simulink model "Q3"  (R2019a)
settings: Solver=FixedStepAuto  StartTime=0.0  StopTime=simulation_stop_time  RelTol=1e-3
values from neighbouring files (symbols this model uses):
  sample_time = 1 / input_sample_freq    (= 1e-06)    [testbench_Q1.m]    (also in testbench_Q3.m; testbench_Q5.m)
libraries: simulink x2
settings Model: Creator=qurai  LastModifiedBy=ASUAD\sasiddi8
settings OptimizationCC: BlockReduction=off  ConditionallyExecuteInputs=off  DefaultParameterBehavior=Inlined
settings DebuggingCC: AlgebraicLoopMsg=error
settings HardwareCC: ProdBitPerPointer=32  ProdBitPerSizeT=32  ProdBitPerPtrDiffT=32  ProdLargestAtomicFloat=None  ProdIntDivRoundTo=Undefined  ProdEndianess=Unspecified  ProdWordSize=32  ProdHWDeviceType=ASIC/FPGA->ASIC/FPGA  TargetBitPerLong=64  TargetBitPerPointer=64  TargetBitPerSizeT=64  TargetBitPerPtrDiffT=64  TargetLongLongMode=on  TargetIntDivRoundTo=Zero  TargetEndianess=LittleEndian  TargetWordSize=64  TargetHWDeviceType=Custom Processor->MATLAB Host Computer  ProdEqTarget=off

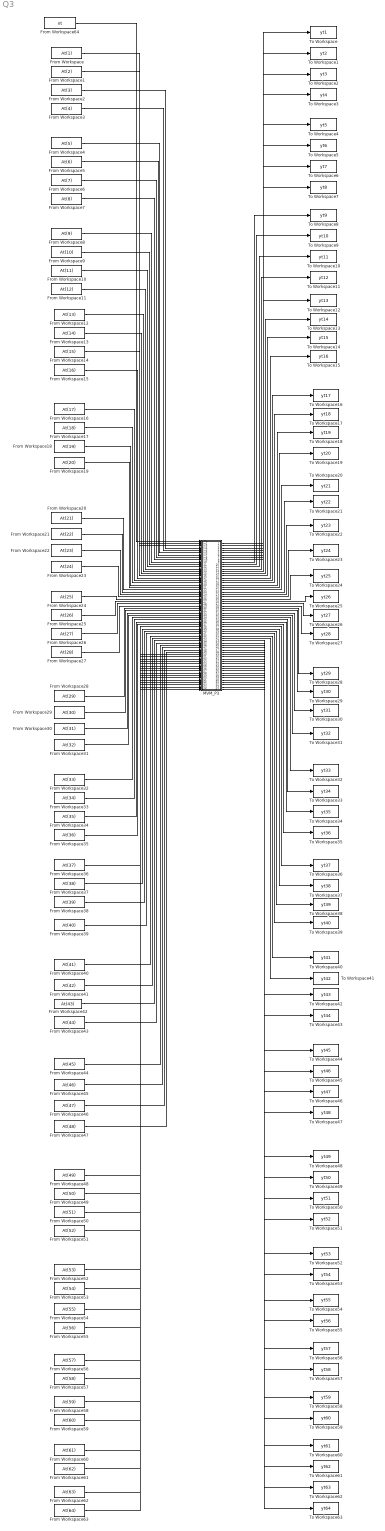
== system Q3 ==
  From Workspace : FromWorkspace  VariableName=At(1)  Interpolate=off  OutputAfterFinalValue=Holding final value
  From Workspace1 : FromWorkspace  VariableName=At(2)  Interpolate=off  OutputAfterFinalValue=Holding final value
  From Workspace10 : FromWorkspace  VariableName=At(11)  Interpolate=off  OutputAfterFinalValue=Holding final value
  From Workspace11 : FromWorkspace  VariableName=At(12)  Interpolate=off  OutputAfterFinalValue=Holding final value
  From Workspace12 : FromWorkspace  VariableName=At(13)  Interpolate=off  OutputAfterFinalValue=Holding final value
  From Workspace13 : FromWorkspace  VariableName=At(14)  Interpolate=off  OutputAfterFinalValue=Holding final value
  From Workspace14 : FromWorkspace  VariableName=At(15)  Interpolate=off  OutputAfterFinalValue=Holding final value
  From Workspace15 : FromWorkspace  VariableName=At(16)  Interpolate=off  OutputAfterFinalValue=Holding final value
  From Workspace16 : FromWorkspace  VariableName=At(17)  Interpolate=off  OutputAfterFinalValue=Holding final value
  From Workspace17 : FromWorkspace  VariableName=At(18)  Interpolate=off  OutputAfterFinalValue=Holding final value
  From Workspace18 : FromWorkspace  VariableName=At(19)  Interpolate=off  OutputAfterFinalValue=Holding final value
  From Workspace19 : FromWorkspace  VariableName=At(20)  Interpolate=off  OutputAfterFinalValue=Holding final value
  From Workspace2 : FromWorkspace  VariableName=At(3)  Interpolate=off  OutputAfterFinalValue=Holding final value
  From Workspace20 : FromWorkspace  VariableName=At(21)  Interpolate=off  OutputAfterFinalValue=Holding final value
  From Workspace21 : FromWorkspace  VariableName=At(22)  Interpolate=off  OutputAfterFinalValue=Holding final value
  From Workspace22 : FromWorkspace  VariableName=At(23)  Interpolate=off  OutputAfterFinalValue=Holding final value
  From Workspace23 : FromWorkspace  VariableName=At(24)  Interpolate=off  OutputAfterFinalValue=Holding final value
  From Workspace24 : FromWorkspace  VariableName=At(25)  Interpolate=off  OutputAfterFinalValue=Holding final value
  From Workspace25 : FromWorkspace  VariableName=At(26)  Interpolate=off  OutputAfterFinalValue=Holding final value
  From Workspace26 : FromWorkspace  VariableName=At(27)  Interpolate=off  OutputAfterFinalValue=Holding final value
  From Workspace27 : FromWorkspace  VariableName=At(28)  Interpolate=off  OutputAfterFinalValue=Holding final value
  From Workspace28 : FromWorkspace  VariableName=At(29)  Interpolate=off  OutputAfterFinalValue=Holding final value
  From Workspace29 : FromWorkspace  VariableName=At(30)  Interpolate=off  OutputAfterFinalValue=Holding final value
  From Workspace3 : FromWorkspace  VariableName=At(4)  Interpolate=off  OutputAfterFinalValue=Holding final value
  From Workspace30 : FromWorkspace  VariableName=At(31)  Interpolate=off  OutputAfterFinalValue=Holding final value
  From Workspace31 : FromWorkspace  VariableName=At(32)  Interpolate=off  OutputAfterFinalValue=Holding final value
  From Workspace32 : FromWorkspace  VariableName=At(33)  Interpolate=off  OutputAfterFinalValue=Holding final value
  From Workspace33 : FromWorkspace  VariableName=At(34)  Interpolate=off  OutputAfterFinalValue=Holding final value
  From Workspace34 : FromWorkspace  VariableName=At(35)  Interpolate=off  OutputAfterFinalValue=Holding final value
  From Workspace35 : FromWorkspace  VariableName=At(36)  Interpolate=off  OutputAfterFinalValue=Holding final value
  From Workspace36 : FromWorkspace  VariableName=At(37)  Interpolate=off  OutputAfterFinalValue=Holding final value
  From Workspace37 : FromWorkspace  VariableName=At(38)  Interpolate=off  OutputAfterFinalValue=Holding final value
  From Workspace38 : FromWorkspace  VariableName=At(39)  Interpolate=off  OutputAfterFinalValue=Holding final value
  From Workspace39 : FromWorkspace  VariableName=At(40)  Interpolate=off  OutputAfterFinalValue=Holding final value
  From Workspace4 : FromWorkspace  VariableName=At(5)  Interpolate=off  OutputAfterFinalValue=Holding final value
  From Workspace40 : FromWorkspace  VariableName=At(41)  Interpolate=off  OutputAfterFinalValue=Holding final value
  From Workspace41 : FromWorkspace  VariableName=At(42)  Interpolate=off  OutputAfterFinalValue=Holding final value
  From Workspace42 : FromWorkspace  VariableName=At(43)  Interpolate=off  OutputAfterFinalValue=Holding final value
  From Workspace43 : FromWorkspace  VariableName=At(44)  Interpolate=off  OutputAfterFinalValue=Holding final value
  From Workspace44 : FromWorkspace  VariableName=At(45)  Interpolate=off  OutputAfterFinalValue=Holding final value
  From Workspace45 : FromWorkspace  VariableName=At(46)  Interpolate=off  OutputAfterFinalValue=Holding final value
  From Workspace46 : FromWorkspace  VariableName=At(47)  Interpolate=off  OutputAfterFinalValue=Holding final value
  From Workspace47 : FromWorkspace  VariableName=At(48)  Interpolate=off  OutputAfterFinalValue=Holding final value
  From Workspace48 : FromWorkspace  VariableName=At(49)  Interpolate=off  OutputAfterFinalValue=Holding final value
  From Workspace49 : FromWorkspace  VariableName=At(50)  Interpolate=off  OutputAfterFinalValue=Holding final value
  From Workspace5 : FromWorkspace  VariableName=At(6)  Interpolate=off  OutputAfterFinalValue=Holding final value
  From Workspace50 : FromWorkspace  VariableName=At(51)  Interpolate=off  OutputAfterFinalValue=Holding final value
  From Workspace51 : FromWorkspace  VariableName=At(52)  Interpolate=off  OutputAfterFinalValue=Holding final value
  From Workspace52 : FromWorkspace  VariableName=At(53)  Interpolate=off  OutputAfterFinalValue=Holding final value
  From Workspace53 : FromWorkspace  VariableName=At(54)  Interpolate=off  OutputAfterFinalValue=Holding final value
  From Workspace54 : FromWorkspace  VariableName=At(55)  Interpolate=off  OutputAfterFinalValue=Holding final value
  From Workspace55 : FromWorkspace  VariableName=At(56)  Interpolate=off  OutputAfterFinalValue=Holding final value
  From Workspace56 : FromWorkspace  VariableName=At(57)  Interpolate=off  OutputAfterFinalValue=Holding final value
  From Workspace57 : FromWorkspace  VariableName=At(58)  Interpolate=off  OutputAfterFinalValue=Holding final value
  From Workspace58 : FromWorkspace  VariableName=At(59)  Interpolate=off  OutputAfterFinalValue=Holding final value
  From Workspace59 : FromWorkspace  VariableName=At(60)  Interpolate=off  OutputAfterFinalValue=Holding final value
  From Workspace6 : FromWorkspace  VariableName=At(7)  Interpolate=off  OutputAfterFinalValue=Holding final value
  From Workspace60 : FromWorkspace  VariableName=At(61)  Interpolate=off  OutputAfterFinalValue=Holding final value
  From Workspace61 : FromWorkspace  VariableName=At(62)  Interpolate=off  OutputAfterFinalValue=Holding final value
  From Workspace62 : FromWorkspace  VariableName=At(63)  Interpolate=off  OutputAfterFinalValue=Holding final value
  From Workspace63 : FromWorkspace  VariableName=At(64)  Interpolate=off  OutputAfterFinalValue=Holding final value
  From Workspace64 : FromWorkspace  VariableName=xt  Interpolate=off  OutputAfterFinalValue=Holding final value
  From Workspace7 : FromWorkspace  VariableName=At(8)  Interpolate=off  OutputAfterFinalValue=Holding final value
  From Workspace8 : FromWorkspace  VariableName=At(9)  Interpolate=off  OutputAfterFinalValue=Holding final value
  From Workspace9 : FromWorkspace  VariableName=At(10)  Interpolate=off  OutputAfterFinalValue=Holding final value
  MVM_P3 : Subsystem  TreatAsAtomicUnit=on  SystemSampleTime=sample_time/16
  To Workspace : ToWorkspace  VariableName=yt1  SaveFormat=Structure With Time  SampleTime=-1
      settings: Save2DSignal=2-D array (concatenate along first dimension)
  To Workspace1 : ToWorkspace  VariableName=yt2  SaveFormat=Structure With Time  SampleTime=-1
      settings: Save2DSignal=2-D array (concatenate along first dimension)
  To Workspace10 : ToWorkspace  VariableName=yt11  SaveFormat=Structure With Time  SampleTime=-1
      settings: Save2DSignal=2-D array (concatenate along first dimension)
  To Workspace11 : ToWorkspace  VariableName=yt12  SaveFormat=Structure With Time  SampleTime=-1
  To Workspace12 : ToWorkspace  VariableName=yt13  SaveFormat=Structure With Time  SampleTime=-1
      settings: Save2DSignal=2-D array (concatenate along first dimension)
  To Workspace13 : ToWorkspace  VariableName=yt14  SaveFormat=Structure With Time  SampleTime=-1
  To Workspace14 : ToWorkspace  VariableName=yt15  SaveFormat=Structure With Time  SampleTime=-1
      settings: Save2DSignal=2-D array (concatenate along first dimension)
  To Workspace15 : ToWorkspace  VariableName=yt16  SaveFormat=Structure With Time  SampleTime=-1
      settings: Save2DSignal=2-D array (concatenate along first dimension)
  To Workspace16 : ToWorkspace  VariableName=yt17  SaveFormat=Structure With Time  SampleTime=-1
      settings: Save2DSignal=2-D array (concatenate along first dimension)
  To Workspace17 : ToWorkspace  VariableName=yt18  SaveFormat=Structure With Time  SampleTime=-1
  To Workspace18 : ToWorkspace  VariableName=yt19  SaveFormat=Structure With Time  SampleTime=-1
      settings: Save2DSignal=2-D array (concatenate along first dimension)
  To Workspace19 : ToWorkspace  VariableName=yt20  SaveFormat=Structure With Time  SampleTime=-1
      settings: Save2DSignal=2-D array (concatenate along first dimension)
  To Workspace2 : ToWorkspace  VariableName=yt3  SaveFormat=Structure With Time  SampleTime=-1
      settings: Save2DSignal=2-D array (concatenate along first dimension)
  To Workspace20 : ToWorkspace  VariableName=yt21  SaveFormat=Structure With Time  SampleTime=-1
      settings: Save2DSignal=2-D array (concatenate along first dimension)
  To Workspace21 : ToWorkspace  VariableName=yt22  SaveFormat=Structure With Time  SampleTime=-1
  To Workspace22 : ToWorkspace  VariableName=yt23  SaveFormat=Structure With Time  SampleTime=-1
      settings: Save2DSignal=2-D array (concatenate along first dimension)
  To Workspace23 : ToWorkspace  VariableName=yt24  SaveFormat=Structure With Time  SampleTime=-1
      settings: Save2DSignal=2-D array (concatenate along first dimension)
  To Workspace24 : ToWorkspace  VariableName=yt25  SaveFormat=Structure With Time  SampleTime=-1
      settings: Save2DSignal=2-D array (concatenate along first dimension)
  To Workspace25 : ToWorkspace  VariableName=yt26  SaveFormat=Structure With Time  SampleTime=-1
  To Workspace26 : ToWorkspace  VariableName=yt27  SaveFormat=Structure With Time  SampleTime=-1
      settings: Save2DSignal=2-D array (concatenate along first dimension)
  To Workspace27 : ToWorkspace  VariableName=yt28  SaveFormat=Structure With Time  SampleTime=-1
      settings: Save2DSignal=2-D array (concatenate along first dimension)
  To Workspace28 : ToWorkspace  VariableName=yt29  SaveFormat=Structure With Time  SampleTime=-1
      settings: Save2DSignal=2-D array (concatenate along first dimension)
  To Workspace29 : ToWorkspace  VariableName=yt30  SaveFormat=Structure With Time  SampleTime=-1
  To Workspace3 : ToWorkspace  VariableName=yt4  SaveFormat=Structure With Time  SampleTime=-1
  To Workspace30 : ToWorkspace  VariableName=yt31  SaveFormat=Structure With Time  SampleTime=-1
      settings: Save2DSignal=2-D array (concatenate along first dimension)
  To Workspace31 : ToWorkspace  VariableName=yt32  SaveFormat=Structure With Time  SampleTime=-1
      settings: Save2DSignal=2-D array (concatenate along first dimension)
  To Workspace32 : ToWorkspace  VariableName=yt33  SaveFormat=Structure With Time  SampleTime=-1
      settings: Save2DSignal=2-D array (concatenate along first dimension)
  To Workspace33 : ToWorkspace  VariableName=yt34  SaveFormat=Structure With Time  SampleTime=-1
  To Workspace34 : ToWorkspace  VariableName=yt35  SaveFormat=Structure With Time  SampleTime=-1
      settings: Save2DSignal=2-D array (concatenate along first dimension)
  To Workspace35 : ToWorkspace  VariableName=yt36  SaveFormat=Structure With Time  SampleTime=-1
      settings: Save2DSignal=2-D array (concatenate along first dimension)
  To Workspace36 : ToWorkspace  VariableName=yt37  SaveFormat=Structure With Time  SampleTime=-1
      settings: Save2DSignal=2-D array (concatenate along first dimension)
  To Workspace37 : ToWorkspace  VariableName=yt38  SaveFormat=Structure With Time  SampleTime=-1
  To Workspace38 : ToWorkspace  VariableName=yt39  SaveFormat=Structure With Time  SampleTime=-1
      settings: Save2DSignal=2-D array (concatenate along first dimension)
  To Workspace39 : ToWorkspace  VariableName=yt40  SaveFormat=Structure With Time  SampleTime=-1
      settings: Save2DSignal=2-D array (concatenate along first dimension)
  To Workspace4 : ToWorkspace  VariableName=yt5  SaveFormat=Structure With Time  SampleTime=-1
      settings: Save2DSignal=2-D array (concatenate along first dimension)
  To Workspace40 : ToWorkspace  VariableName=yt41  SaveFormat=Structure With Time  SampleTime=-1
      settings: Save2DSignal=2-D array (concatenate along first dimension)
  To Workspace41 : ToWorkspace  VariableName=yt42  SaveFormat=Structure With Time  SampleTime=-1
  To Workspace42 : ToWorkspace  VariableName=yt43  SaveFormat=Structure With Time  SampleTime=-1
      settings: Save2DSignal=2-D array (concatenate along first dimension)
  To Workspace43 : ToWorkspace  VariableName=yt44  SaveFormat=Structure With Time  SampleTime=-1
      settings: Save2DSignal=2-D array (concatenate along first dimension)
  To Workspace44 : ToWorkspace  VariableName=yt45  SaveFormat=Structure With Time  SampleTime=-1
      settings: Save2DSignal=2-D array (concatenate along first dimension)
  To Workspace45 : ToWorkspace  VariableName=yt46  SaveFormat=Structure With Time  SampleTime=-1
  To Workspace46 : ToWorkspace  VariableName=yt47  SaveFormat=Structure With Time  SampleTime=-1
      settings: Save2DSignal=2-D array (concatenate along first dimension)
  To Workspace47 : ToWorkspace  VariableName=yt48  SaveFormat=Structure With Time  SampleTime=-1
      settings: Save2DSignal=2-D array (concatenate along first dimension)
  To Workspace48 : ToWorkspace  VariableName=yt49  SaveFormat=Structure With Time  SampleTime=-1
      settings: Save2DSignal=2-D array (concatenate along first dimension)
  To Workspace49 : ToWorkspace  VariableName=yt50  SaveFormat=Structure With Time  SampleTime=-1
  To Workspace5 : ToWorkspace  VariableName=yt6  SaveFormat=Structure With Time  SampleTime=-1
      settings: Save2DSignal=2-D array (concatenate along first dimension)
  To Workspace50 : ToWorkspace  VariableName=yt51  SaveFormat=Structure With Time  SampleTime=-1
      settings: Save2DSignal=2-D array (concatenate along first dimension)
  To Workspace51 : ToWorkspace  VariableName=yt52  SaveFormat=Structure With Time  SampleTime=-1
      settings: Save2DSignal=2-D array (concatenate along first dimension)
  To Workspace52 : ToWorkspace  VariableName=yt53  SaveFormat=Structure With Time  SampleTime=-1
      settings: Save2DSignal=2-D array (concatenate along first dimension)
  To Workspace53 : ToWorkspace  VariableName=yt54  SaveFormat=Structure With Time  SampleTime=-1
  To Workspace54 : ToWorkspace  VariableName=yt55  SaveFormat=Structure With Time  SampleTime=-1
      settings: Save2DSignal=2-D array (concatenate along first dimension)
  To Workspace55 : ToWorkspace  VariableName=yt56  SaveFormat=Structure With Time  SampleTime=-1
      settings: Save2DSignal=2-D array (concatenate along first dimension)
  To Workspace56 : ToWorkspace  VariableName=yt57  SaveFormat=Structure With Time  SampleTime=-1
      settings: Save2DSignal=2-D array (concatenate along first dimension)
  To Workspace57 : ToWorkspace  VariableName=yt58  SaveFormat=Structure With Time  SampleTime=-1
  To Workspace58 : ToWorkspace  VariableName=yt59  SaveFormat=Structure With Time  SampleTime=-1
      settings: Save2DSignal=2-D array (concatenate along first dimension)
  To Workspace59 : ToWorkspace  VariableName=yt60  SaveFormat=Structure With Time  SampleTime=-1
      settings: Save2DSignal=2-D array (concatenate along first dimension)
  To Workspace6 : ToWorkspace  VariableName=yt7  SaveFormat=Structure With Time  SampleTime=-1
      settings: Save2DSignal=2-D array (concatenate along first dimension)
  To Workspace60 : ToWorkspace  VariableName=yt61  SaveFormat=Structure With Time  SampleTime=-1
      settings: Save2DSignal=2-D array (concatenate along first dimension)
  To Workspace61 : ToWorkspace  VariableName=yt62  SaveFormat=Structure With Time  SampleTime=-1
  To Workspace62 : ToWorkspace  VariableName=yt63  SaveFormat=Structure With Time  SampleTime=-1
      settings: Save2DSignal=2-D array (concatenate along first dimension)
  To Workspace63 : ToWorkspace  VariableName=yt64  SaveFormat=Structure With Time  SampleTime=-1
      settings: Save2DSignal=2-D array (concatenate along first dimension)
  To Workspace7 : ToWorkspace  VariableName=yt8  SaveFormat=Structure With Time  SampleTime=-1
  To Workspace8 : ToWorkspace  VariableName=yt9  SaveFormat=Structure With Time  SampleTime=-1
      settings: Save2DSignal=2-D array (concatenate along first dimension)
  To Workspace9 : ToWorkspace  VariableName=yt10  SaveFormat=Structure With Time  SampleTime=-1
      settings: Save2DSignal=2-D array (concatenate along first dimension)
  wires:
  From Workspace64/1 -> MVM_P3/1(In1)
  From Workspace/1 -> MVM_P3/2(In2)
  From Workspace1/1 -> MVM_P3/3(In3)
  From Workspace2/1 -> MVM_P3/4(In4)
  From Workspace3/1 -> MVM_P3/5(In5)
  From Workspace4/1 -> MVM_P3/6(In6)
  From Workspace5/1 -> MVM_P3/7(In7)
  From Workspace6/1 -> MVM_P3/8(In8)
  From Workspace7/1 -> MVM_P3/9(In9)
  From Workspace8/1 -> MVM_P3/10(In10)
  From Workspace9/1 -> MVM_P3/11(In11)
  From Workspace10/1 -> MVM_P3/12(In12)
  From Workspace11/1 -> MVM_P3/13(In13)
  From Workspace12/1 -> MVM_P3/14(In14)
  From Workspace13/1 -> MVM_P3/15(In15)
  From Workspace14/1 -> MVM_P3/16(In16)
  From Workspace15/1 -> MVM_P3/17(In17)
  From Workspace16/1 -> MVM_P3/18(In18)
  From Workspace17/1 -> MVM_P3/19(In19)
  From Workspace18/1 -> MVM_P3/20(In20)
  From Workspace19/1 -> MVM_P3/21(In21)
  From Workspace20/1 -> MVM_P3/22(In22)
  From Workspace21/1 -> MVM_P3/23(In23)
  From Workspace22/1 -> MVM_P3/24(In24)
  From Workspace23/1 -> MVM_P3/25(In25)
  From Workspace24/1 -> MVM_P3/26(In26)
  From Workspace25/1 -> MVM_P3/27(In27)
  From Workspace26/1 -> MVM_P3/28(In28)
  From Workspace27/1 -> MVM_P3/29(In29)
  From Workspace28/1 -> MVM_P3/30(In30)
  From Workspace29/1 -> MVM_P3/31(In31)
  From Workspace30/1 -> MVM_P3/32(In32)
  From Workspace31/1 -> MVM_P3/33(In33)
  From Workspace32/1 -> MVM_P3/34(In34)
  From Workspace33/1 -> MVM_P3/35(In35)
  From Workspace34/1 -> MVM_P3/36(In36)
  From Workspace35/1 -> MVM_P3/37(In37)
  From Workspace36/1 -> MVM_P3/38(In38)
  From Workspace37/1 -> MVM_P3/39(In39)
  From Workspace38/1 -> MVM_P3/40(In40)
  From Workspace39/1 -> MVM_P3/41(In41)
  From Workspace40/1 -> MVM_P3/42(In42)
  From Workspace41/1 -> MVM_P3/43(In43)
  From Workspace42/1 -> MVM_P3/44(In44)
  From Workspace43/1 -> MVM_P3/45(In45)
  From Workspace44/1 -> MVM_P3/46(In46)
  From Workspace45/1 -> MVM_P3/47(In47)
  From Workspace46/1 -> MVM_P3/48(In48)
  From Workspace47/1 -> MVM_P3/49(In49)
  From Workspace48/1 -> MVM_P3/50(In50)
  From Workspace49/1 -> MVM_P3/51(In51)
  From Workspace50/1 -> MVM_P3/52(In52)
  From Workspace51/1 -> MVM_P3/53(In53)
  From Workspace52/1 -> MVM_P3/54(In54)
  From Workspace53/1 -> MVM_P3/55(In55)
  From Workspace54/1 -> MVM_P3/56(In56)
  From Workspace55/1 -> MVM_P3/57(In57)
  From Workspace56/1 -> MVM_P3/58(In58)
  From Workspace57/1 -> MVM_P3/59(In59)
  From Workspace58/1 -> MVM_P3/60(In60)
  From Workspace59/1 -> MVM_P3/61(In61)
  From Workspace60/1 -> MVM_P3/62(In62)
  From Workspace61/1 -> MVM_P3/63(In63)
  From Workspace62/1 -> MVM_P3/64(In64)
  From Workspace63/1 -> MVM_P3/65(In65)
  MVM_P3/1(Out1) -> To Workspace/1
  MVM_P3/2(Out2) -> To Workspace1/1
  MVM_P3/3(Out3) -> To Workspace2/1
  MVM_P3/4(Out4) -> To Workspace3/1
  MVM_P3/5(Out5) -> To Workspace4/1
  MVM_P3/6(Out6) -> To Workspace5/1
  MVM_P3/7(Out7) -> To Workspace6/1
  MVM_P3/8(Out8) -> To Workspace7/1
  MVM_P3/9(Out9) -> To Workspace8/1
  MVM_P3/10(Out10) -> To Workspace9/1
  MVM_P3/11(Out11) -> To Workspace10/1
  MVM_P3/12(Out12) -> To Workspace11/1
  MVM_P3/13(Out13) -> To Workspace12/1
  MVM_P3/14(Out14) -> To Workspace13/1
  MVM_P3/15(Out15) -> To Workspace14/1
  MVM_P3/16(Out16) -> To Workspace15/1
  MVM_P3/17(Out17) -> To Workspace16/1
  MVM_P3/18(Out18) -> To Workspace17/1
  MVM_P3/19(Out19) -> To Workspace18/1
  MVM_P3/20(Out20) -> To Workspace19/1
  MVM_P3/21(Out21) -> To Workspace20/1
  MVM_P3/22(Out22) -> To Workspace21/1
  MVM_P3/23(Out23) -> To Workspace22/1
  MVM_P3/24(Out24) -> To Workspace23/1
  MVM_P3/25(Out25) -> To Workspace24/1
  MVM_P3/26(Out26) -> To Workspace25/1
  MVM_P3/27(Out27) -> To Workspace26/1
  MVM_P3/28(Out28) -> To Workspace27/1
  MVM_P3/29(Out29) -> To Workspace28/1
  MVM_P3/30(Out30) -> To Workspace29/1
  MVM_P3/31(Out31) -> To Workspace30/1
  MVM_P3/32(Out32) -> To Workspace31/1
  MVM_P3/33(Out33) -> To Workspace32/1
  MVM_P3/34(Out34) -> To Workspace33/1
  MVM_P3/35(Out35) -> To Workspace34/1
  MVM_P3/36(Out36) -> To Workspace35/1
  MVM_P3/37(Out37) -> To Workspace36/1
  MVM_P3/38(Out38) -> To Workspace37/1
  MVM_P3/39(Out39) -> To Workspace38/1
  MVM_P3/40(Out40) -> To Workspace39/1
  MVM_P3/41(Out41) -> To Workspace40/1
  MVM_P3/42(Out42) -> To Workspace41/1
  MVM_P3/43(Out43) -> To Workspace42/1
  MVM_P3/44(Out44) -> To Workspace43/1
  MVM_P3/45(Out45) -> To Workspace44/1
  MVM_P3/46(Out46) -> To Workspace45/1
  MVM_P3/47(Out47) -> To Workspace46/1
  MVM_P3/48(Out48) -> To Workspace47/1
  MVM_P3/49(Out49) -> To Workspace48/1
  MVM_P3/50(Out50) -> To Workspace49/1
  MVM_P3/51(Out51) -> To Workspace50/1
  MVM_P3/52(Out52) -> To Workspace51/1
  MVM_P3/53(Out53) -> To Workspace52/1
  MVM_P3/54(Out54) -> To Workspace53/1
  MVM_P3/55(Out55) -> To Workspace54/1
  MVM_P3/56(Out56) -> To Workspace55/1
  MVM_P3/57(Out57) -> To Workspace56/1
  MVM_P3/58(Out58) -> To Workspace57/1
  MVM_P3/59(Out59) -> To Workspace58/1
  MVM_P3/60(Out60) -> To Workspace59/1
  MVM_P3/61(Out61) -> To Workspace60/1
  MVM_P3/62(Out62) -> To Workspace61/1
  MVM_P3/63(Out63) -> To Workspace62/1
  MVM_P3/64(Out64) -> To Workspace63/1

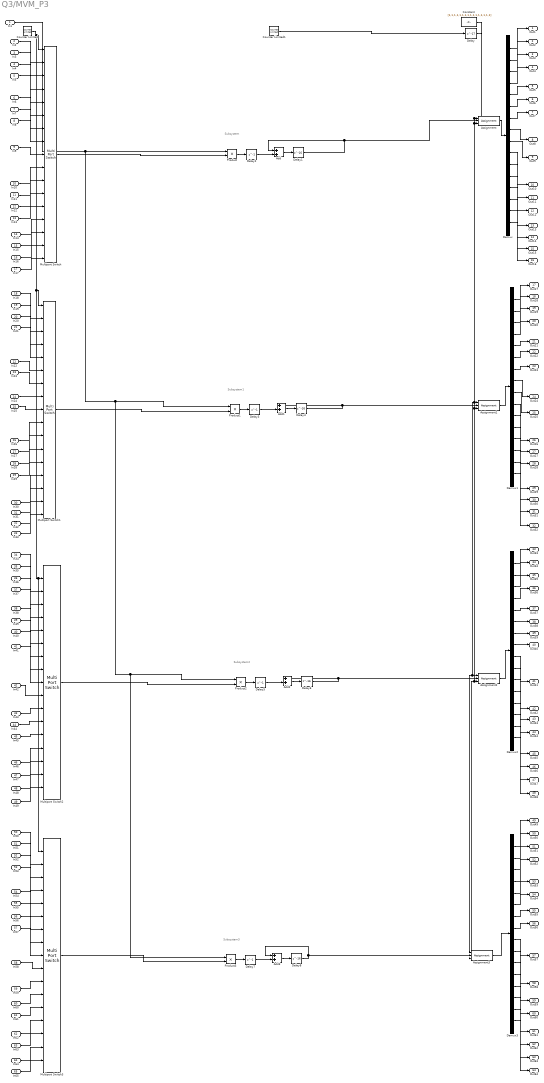
== system Q3/MVM_P3 ==
  note: Subsystem3
  note: Subsystem2
  note: Subsystem1
  note: Subsystem
  In1 : Inport
  In2 : Inport  Port=2
  In3 : Inport  Port=3
  In4 : Inport  Port=4
  In5 : Inport  Port=5
  In6 : Inport  Port=6
  In7 : Inport  Port=7
  In8 : Inport  Port=8
  In9 : Inport  Port=9
  In10 : Inport  Port=10
  In11 : Inport  Port=11
  In12 : Inport  Port=12
  In13 : Inport  Port=13
  In14 : Inport  Port=14
  In15 : Inport  Port=15
  In16 : Inport  Port=16
  In17 : Inport  Port=17
  In18 : Inport  Port=18
  In19 : Inport  Port=19
  In20 : Inport  Port=20
  In21 : Inport  Port=21
  In22 : Inport  Port=22
  In23 : Inport  Port=23
  In24 : Inport  Port=24
  In25 : Inport  Port=25
  In26 : Inport  Port=26
  In27 : Inport  Port=27
  In28 : Inport  Port=28
  In29 : Inport  Port=29
  In30 : Inport  Port=30
  In31 : Inport  Port=31
  In32 : Inport  Port=32
  In33 : Inport  Port=33
  In34 : Inport  Port=34
  In35 : Inport  Port=35
  In36 : Inport  Port=36
  In37 : Inport  Port=37
  In38 : Inport  Port=38
  In39 : Inport  Port=39
  In40 : Inport  Port=40
  In41 : Inport  Port=41
  In42 : Inport  Port=42
  In43 : Inport  Port=43
  In44 : Inport  Port=44
  In45 : Inport  Port=45
  In46 : Inport  Port=46
  In47 : Inport  Port=47
  In48 : Inport  Port=48
  In49 : Inport  Port=49
  In50 : Inport  Port=50
  In51 : Inport  Port=51
  In52 : Inport  Port=52
  In53 : Inport  Port=53
  In54 : Inport  Port=54
  In55 : Inport  Port=55
  In56 : Inport  Port=56
  In57 : Inport  Port=57
  In58 : Inport  Port=58
  In59 : Inport  Port=59
  In60 : Inport  Port=60
  In61 : Inport  Port=61
  In62 : Inport  Port=62
  In63 : Inport  Port=63
  In64 : Inport  Port=64
  In65 : Inport  Port=65
  Add{,1..3} (4 alike) : Sum
  Assignment{,1..3} (4 alike) : Assignment  IndexMode=Zero-based  IndexOptions=Starting index (port)  Indices=1  OutputSizes=1
  Constant : Constant  Value=[1,1,1,1,1,1,1,1,1,1,1,1,1,1,1,1]  SampleTime=6.25e-8
  Counter Limited : simulink/Sources/Counter Limited  uplimit=15  tsamp=6.25e-8
  Counter Limited1 : simulink/Sources/Counter Limited  uplimit=15  tsamp=6.25e-8
  Delay : Delay  DelayLength=17  InitialCondition=0  SampleTime=6.25e-8
  Delay{1,4,6,8} (4 alike) : Delay  DelayLength=16  InitialCondition=0
  Delay{2..3,5,7} (4 alike) : Delay  DelayLength=1  InitialCondition=0
  Demux{,1..3} (4 alike) : Demux  Outputs=16
  Multiport Switch{,1..3} (4 alike) : MultiPortSwitch  DataPortOrder=Zero-based contiguous  Inputs=16  zeroidx=on
  Product{,1..3} (4 alike) : Product
  Out1 : Outport
  Out2 : Outport  Port=2
  Out3 : Outport  Port=3
  Out4 : Outport  Port=4
  Out5 : Outport  Port=5
  Out6 : Outport  Port=6
  Out7 : Outport  Port=7
  Out8 : Outport  Port=8
  Out9 : Outport  Port=9
  Out10 : Outport  Port=10
  Out11 : Outport  Port=11
  Out12 : Outport  Port=12
  Out13 : Outport  Port=13
  Out14 : Outport  Port=14
  Out15 : Outport  Port=15
  Out16 : Outport  Port=16
  Out17 : Outport  Port=17
  Out18 : Outport  Port=18
  Out19 : Outport  Port=19
  Out20 : Outport  Port=20
  Out21 : Outport  Port=21
  Out22 : Outport  Port=22
  Out23 : Outport  Port=23
  Out24 : Outport  Port=24
  Out25 : Outport  Port=25
  Out26 : Outport  Port=26
  Out27 : Outport  Port=27
  Out28 : Outport  Port=28
  Out29 : Outport  Port=29
  Out30 : Outport  Port=30
  Out31 : Outport  Port=31
  Out32 : Outport  Port=32
  Out33 : Outport  Port=33
  Out34 : Outport  Port=34
  Out35 : Outport  Port=35
  Out36 : Outport  Port=36
  Out37 : Outport  Port=37
  Out38 : Outport  Port=38
  Out39 : Outport  Port=39
  Out40 : Outport  Port=40
  Out41 : Outport  Port=41
  Out42 : Outport  Port=42
  Out43 : Outport  Port=43
  Out44 : Outport  Port=44
  Out45 : Outport  Port=45
  Out46 : Outport  Port=46
  Out47 : Outport  Port=47
  Out48 : Outport  Port=48
  Out49 : Outport  Port=49
  Out50 : Outport  Port=50
  Out51 : Outport  Port=51
  Out52 : Outport  Port=52
  Out53 : Outport  Port=53
  Out54 : Outport  Port=54
  Out55 : Outport  Port=55
  Out56 : Outport  Port=56
  Out57 : Outport  Port=57
  Out58 : Outport  Port=58
  Out59 : Outport  Port=59
  Out60 : Outport  Port=60
  Out61 : Outport  Port=61
  Out62 : Outport  Port=62
  Out63 : Outport  Port=63
  Out64 : Outport  Port=64
  wires:
  Demux2/4 -> Out36/1
  In62/1 -> Multiport Switch3/14
  Demux3/1 -> Out49/1
  In53/1 -> Multiport Switch3/5
  In26/1 -> Multiport Switch1/10
  Demux3/13 -> Out61/1
  In21/1 -> Multiport Switch1/5
  Demux2/14 -> Out46/1
  Demux2/1 -> Out33/1
  Demux2/12 -> Out44/1
  In40/1 -> Multiport Switch2/8
  Demux1/5 -> Out21/1
  Demux3/8 -> Out56/1
  Demux2/11 -> Out43/1
  Demux/12 -> Out12/1
  Demux/16 -> Out16/1
  Demux1/6 -> Out22/1
  In60/1 -> Multiport Switch3/12
  In10/1 -> Multiport Switch/10
  In33/1 -> Multiport Switch1/17
  In25/1 -> Multiport Switch1/9
  In28/1 -> Multiport Switch1/12
  Demux2/7 -> Out39/1
  Demux1/7 -> Out23/1
  Demux/10 -> Out10/1
  In48/1 -> Multiport Switch2/16
  In22/1 -> Multiport Switch1/6
  Demux3/4 -> Out52/1
  Demux1/2 -> Out18/1
  Demux/14 -> Out14/1
  Demux1/10 -> Out26/1
  In23/1 -> Multiport Switch1/7
  In50/1 -> Multiport Switch3/2
  Demux2/5 -> Out37/1
  In56/1 -> Multiport Switch3/8
  In57/1 -> Multiport Switch3/9
  Demux1/16 -> Out32/1
  In43/1 -> Multiport Switch2/11
  Demux2/2 -> Out34/1
  In39/1 -> Multiport Switch2/7
  In18/1 -> Multiport Switch1/2
  Demux3/14 -> Out62/1
  In55/1 -> Multiport Switch3/7
  In46/1 -> Multiport Switch2/14
  Delay4/1 -> Assignment1/2, Add1/1
  In34/1 -> Multiport Switch2/2
  Demux3/16 -> Out64/1
  Demux2/13 -> Out45/1
  In64/1 -> Multiport Switch3/16
  In38/1 -> Multiport Switch2/6
  Delay/1 -> Assignment3/3, Assignment2/3, Assignment1/3, Assignment/3
  In37/1 -> Multiport Switch2/5
  In61/1 -> Multiport Switch3/13
  In54/1 -> Multiport Switch3/6
  Demux2/15 -> Out47/1
  In31/1 -> Multiport Switch1/15
  In45/1 -> Multiport Switch2/13
  Demux3/12 -> Out60/1
  Assignment/1 -> Demux/1
  In35/1 -> Multiport Switch2/3
  In24/1 -> Multiport Switch1/8
  In16/1 -> Multiport Switch/16
  Demux/6 -> Out6/1
  Demux3/11 -> Out59/1
  In8/1 -> Multiport Switch/8
  In5/1 -> Multiport Switch/5
  Demux/15 -> Out15/1
  In32/1 -> Multiport Switch1/16
  Demux1/11 -> Out27/1
  Demux1/14 -> Out30/1
  In42/1 -> Multiport Switch2/10
  In63/1 -> Multiport Switch3/15
  Demux2/6 -> Out38/1
  Demux1/8 -> Out24/1
  Demux1/13 -> Out29/1
  Demux1/3 -> Out19/1
  In11/1 -> Multiport Switch/11
  In58/1 -> Multiport Switch3/10
  Counter Limited1/1 -> Delay/1
  In15/1 -> Multiport Switch/15
  Demux/8 -> Out8/1
  In27/1 -> Multiport Switch1/11
  In6/1 -> Multiport Switch/6
  Demux/9 -> Out9/1
  Constant/1 -> Assignment3/1, Assignment2/1, Assignment1/1, Assignment/1
  In9/1 -> Multiport Switch/9
  Demux2/8 -> Out40/1
  In59/1 -> Multiport Switch3/11
  In20/1 -> Multiport Switch1/4
  Demux1/4 -> Out20/1
  In65/1 -> Multiport Switch3/17
  Delay1/1 -> Assignment/2, Add/1
  In12/1 -> Multiport Switch/12
  Counter Limited/1 -> Multiport Switch/1, Multiport Switch3/1, Multiport Switch2/1, Multiport Switch1/1
  In44/1 -> Multiport Switch2/12
  Delay8/1 -> Assignment3/2, Add3/1
  Demux/7 -> Out7/1
  In51/1 -> Multiport Switch3/3
  Demux/11 -> Out11/1
  Delay6/1 -> Assignment2/2, Add2/1
  Demux2/9 -> Out41/1
  Assignment2/1 -> Demux2/1
  Demux3/6 -> Out54/1
  Demux1/12 -> Out28/1
  Demux/4 -> Out4/1
  Demux2/16 -> Out48/1
  Demux/1 -> Out1/1
  Demux1/1 -> Out17/1
  Demux3/5 -> Out53/1
  Demux3/15 -> Out63/1
  In4/1 -> Multiport Switch/4
  Demux1/9 -> Out25/1
  Demux3/3 -> Out51/1
  In7/1 -> Multiport Switch/7
  Assignment1/1 -> Demux1/1
  Demux3/10 -> Out58/1
  Demux/3 -> Out3/1
  Demux3/2 -> Out50/1
  In2/1 -> Multiport Switch/2
  Demux/5 -> Out5/1
  In29/1 -> Multiport Switch1/13
  In14/1 -> Multiport Switch/14
  Demux3/7 -> Out55/1
  In30/1 -> Multiport Switch1/14
  In41/1 -> Multiport Switch2/9
  In19/1 -> Multiport Switch1/3
  Demux3/9 -> Out57/1
  Assignment3/1 -> Demux3/1
  In36/1 -> Multiport Switch2/4
  Demux/2 -> Out2/1
  Demux2/3 -> Out35/1
  Demux1/15 -> Out31/1
  In3/1 -> Multiport Switch/3
  Demux2/10 -> Out42/1
  In47/1 -> Multiport Switch2/15
  In52/1 -> Multiport Switch3/4
  In17/1 -> Multiport Switch/17
  In13/1 -> Multiport Switch/13
  In49/1 -> Multiport Switch2/17
  Demux/13 -> Out13/1
  Multiport Switch/1 -> Product/2
  Product/1 -> Delay2/1
  Delay2/1 -> Add/2
  Add/1 -> Delay1/1
  Multiport Switch1/1 -> Product1/2
  Product1/1 -> Delay3/1
  Delay3/1 -> Add1/2
  Add1/1 -> Delay4/1
  Multiport Switch2/1 -> Product2/2
  Product2/1 -> Delay5/1
  Delay5/1 -> Add2/2
  Add2/1 -> Delay6/1
  Multiport Switch3/1 -> Product3/2
  Product3/1 -> Delay7/1
  Delay7/1 -> Add3/2
  In1/1 -> Product/1, Product1/1, Product3/1, Product2/1
  Add3/1 -> Delay8/1
